simulink model "ArryManipulation"  (R2021a)
settings: Solver=FixedStepDiscrete  StartTime=0.0  StopTime=20  FixedStep=0.1  RelTol=1e-3
settings Model: Creator=mymind  LastModifiedBy=mymind

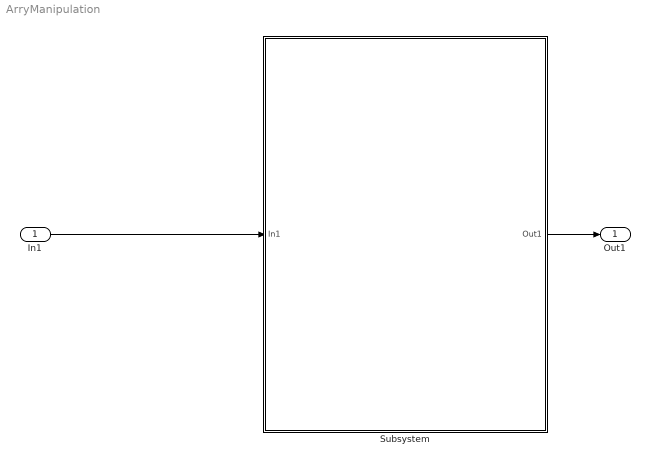
== system ArryManipulation ==
  In1 : Inport
  Subsystem : Subsystem  TreatAsAtomicUnit=on
  Out1 : Outport
  wires:
  In1/1 -> Subsystem/1(In1)
  Subsystem/1(Out1) -> Out1/1

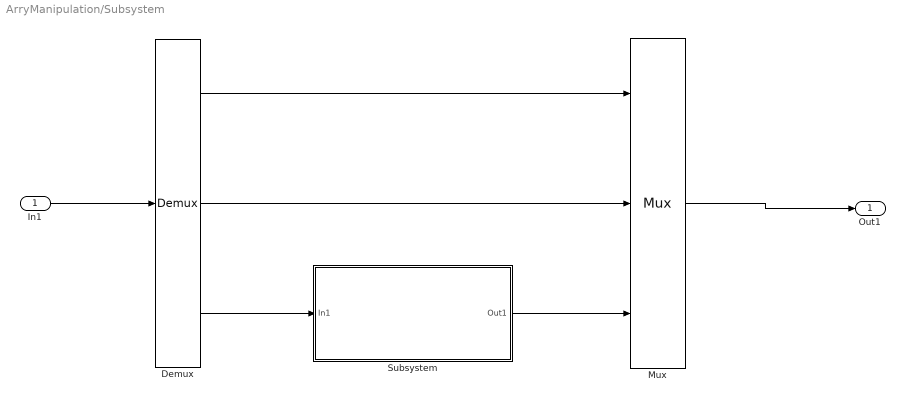
== system ArryManipulation/Subsystem ==
  In1 : Inport
  Demux : Demux  Outputs=3
  Mux : Mux  Inputs=3
  Subsystem : Subsystem
  Out1 : Outport
  wires:
  Mux/1 -> Out1/1
  In1/1 -> Demux/1
  Demux/1 -> Mux/1
  Demux/2 -> Mux/2
  Demux/3 -> Subsystem/1(In1)
  Subsystem/1(Out1) -> Mux/3

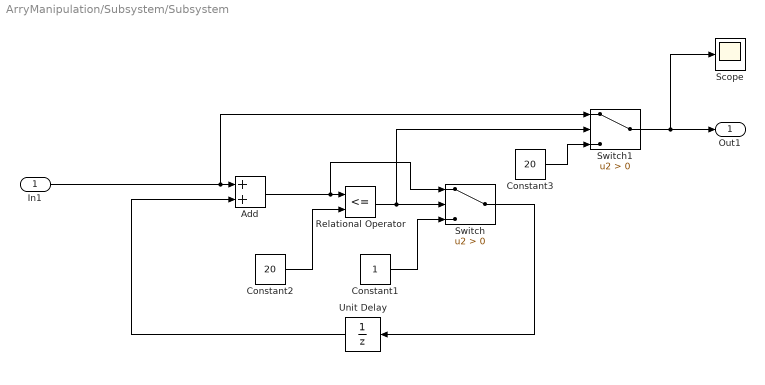
== system ArryManipulation/Subsystem/Subsystem ==
  In1 : Inport
  Add : Sum
  Constant1 : Constant
  Constant2 : Constant  Value=20
  Constant3 : Constant  Value=20
  Relational Operator : RelationalOperator  Operator=<=  OutDataTypeStr=boolean  RndMeth=Simplest
  Scope : Scope
  Switch : Switch  Criteria=u2 > Threshold
  Switch1 : Switch  Criteria=u2 > Threshold
  Unit Delay : UnitDelay  SampleTime=-1  HasFrameUpgradeWarning=on
  Out1 : Outport
  wires:
  In1/1 -> Switch1/1, Add/1
  Constant2/1 -> Relational Operator/2
  Unit Delay/1 -> Add/2
  Add/1 -> Switch/1, Relational Operator/1
  Relational Operator/1 -> Switch/2, Switch1/2
  Constant1/1 -> Switch/3
  Switch/1 -> Unit Delay/1
  Switch1/1 -> Scope/1, Out1/1
  Constant3/1 -> Switch1/3
